simulink model "DiscreteSF_latest"  (R2019b)
settings: Solver=VariableStepAuto  StartTime=0.0  StopTime=1500  RelTol=1e-3
values from neighbouring files (symbols this model uses):
  A3 = [1 -49.59 4.877; 0 0.9835 0; 0 0 0.9512]    [DiscreteSystem.m]
  A3_c = [0 -th2 th4; 0 -1/th3 0; 0 0 -1/th5]    [DiscreteSystem.m]
  A5 = [1 -49.59 -0.4121 4.877 0.1209; 0 0.9835 0.01639 0 0; 0 0 0.9835 0 0 ... (first row only)    [DiscreteSystem.m]
  B3 = [0.85 -0.4144 0.1229; 0 0.01653 0; 0 0 0.04877]    [DiscreteSystem.m]
  B3_c = [th1 0 0; 0 1/th3 0; 0 0 1/th5]    [DiscreteSystem.m]
  B5 = [0.85 -0.002296 0.002032; 0 0.0001374 0; 0 0.01653 0; 0 0 0.001209 ... (first row only)    [DiscreteSystem.m]
  C3 = [1 0 0; 0 1 0; 0 0 1]    [DiscreteSystem.m]
  C3_c = [1 0 0; 0 1 0; 0 0 1]    [DiscreteSystem.m]
  C5 = [1 0 0 0 0; 0 1 0 0 0; 0 0 1 0 0; 0 0 0 1 0; 0 0 0 0 1]    [DiscreteSystem.m]
  D3 = [0 0 0; 0 0 0; 0 0 0]    [DiscreteSystem.m]
  D3_c = [0 0 0; 0 0 0; 0 0 0]    [DiscreteSystem.m]
  D5 = [0 0 0; 0 0 0; 0 0 0; 0 0 0; 0 0 0]    [DiscreteSystem.m]
  F3 = [k/th2 -k*th3 (k*th5*th4)/(th2)]    [DiscreteSystem.m]
  F5 = k*[1/th2 -th3 -th3 (th4*th5)/th2 (th4*th5)/th2]    [DiscreteSystem.m]
  L = [1.05; 0; 0; 0; 0]    [DiscreteSystem.m]
  th1 = 0.85    [DiscreteSystem.m]
  th2 = 50    [DiscreteSystem.m]
  th3 = 60    [DiscreteSystem.m]
undefined symbols (not defined in the file or in its folder): C
libraries: dspsrcs4 x3
settings Model: Creator=akshita_jain  LastModifiedBy=akshita_jain

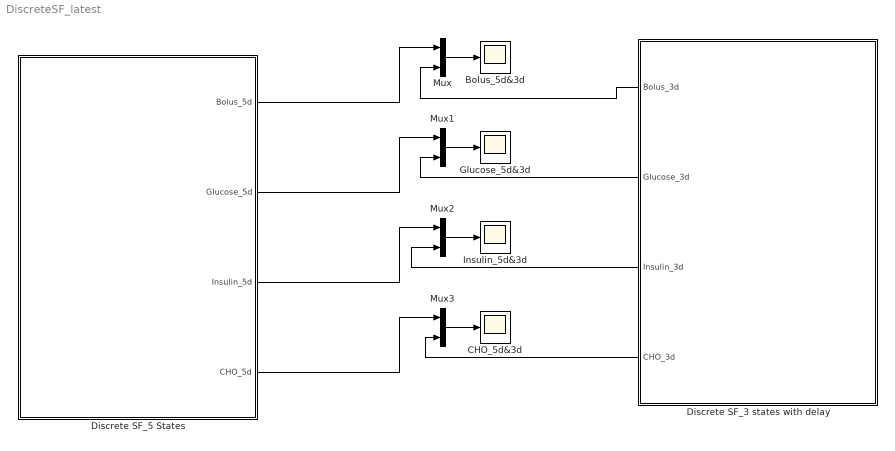
== system DiscreteSF_latest ==
  Bolus_5d&3d : Scope
  CHO_5d&3d : Scope
  Discrete SF_3 states with delay : Subsystem
  Discrete SF_5 States : Subsystem
  Glucose_5d&3d : Scope
  Insulin_5d&3d : Scope
  Mux{,1..3} (4 alike) : Mux  Inputs=2
  wires:
  Discrete SF_5 States/1(Bolus_5d) -> Mux/1
  Discrete SF_3 states with delay/1(Bolus_3d) -> Mux/2
  Mux/1 -> Bolus_5d&3d/1
  Mux1/1 -> Glucose_5d&3d/1
  Discrete SF_5 States/2(Glucose_5d) -> Mux1/1
  Discrete SF_3 states with delay/2(Glucose_3d) -> Mux1/2
  Mux2/1 -> Insulin_5d&3d/1
  Discrete SF_5 States/3(Insulin_5d) -> Mux2/1
  Discrete SF_3 states with delay/3(Insulin_3d) -> Mux2/2
  Discrete SF_5 States/4(CHO_5d) -> Mux3/1
  Mux3/1 -> CHO_5d&3d/1
  Discrete SF_3 states with delay/4(CHO_3d) -> Mux3/2

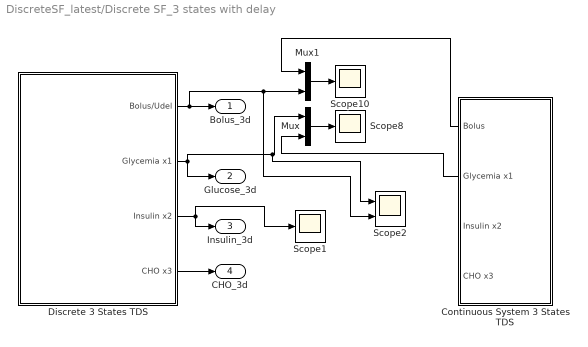
== system DiscreteSF_latest/Discrete SF_3 states with delay ==
  Continuous System 3 States TDS : Subsystem
  Discrete 3 States TDS : Subsystem
  Mux : Mux  Inputs=2
  Mux1 : Mux  Inputs=2
  Scope1 : Scope
  Scope10 : Scope
  Scope2 : Scope  NumInputPorts=2
  Scope8 : Scope
  Bolus_3d : Outport
  Glucose_3d : Outport  Port=2
  Insulin_3d : Outport  Port=3
  CHO_3d : Outport  Port=4
  wires:
  Discrete 3 States TDS/2(Glycemia x1) -> Glucose_3d/1, Scope2/1, Mux/1
  Discrete 3 States TDS/3(Insulin x2) -> Insulin_3d/1, Scope1/1
  Discrete 3 States TDS/4(CHO x3) -> CHO_3d/1
  Continuous System 3 States TDS/1(Bolus) -> Mux1/1
  Continuous System 3 States TDS/2(Glycemia x1) -> Mux/2
  Mux/1 -> Scope8/1
  Mux1/1 -> Scope10/1
  Discrete 3 States TDS/1(Bolus/Udel) -> Bolus_3d/1, Scope2/2, Mux1/2

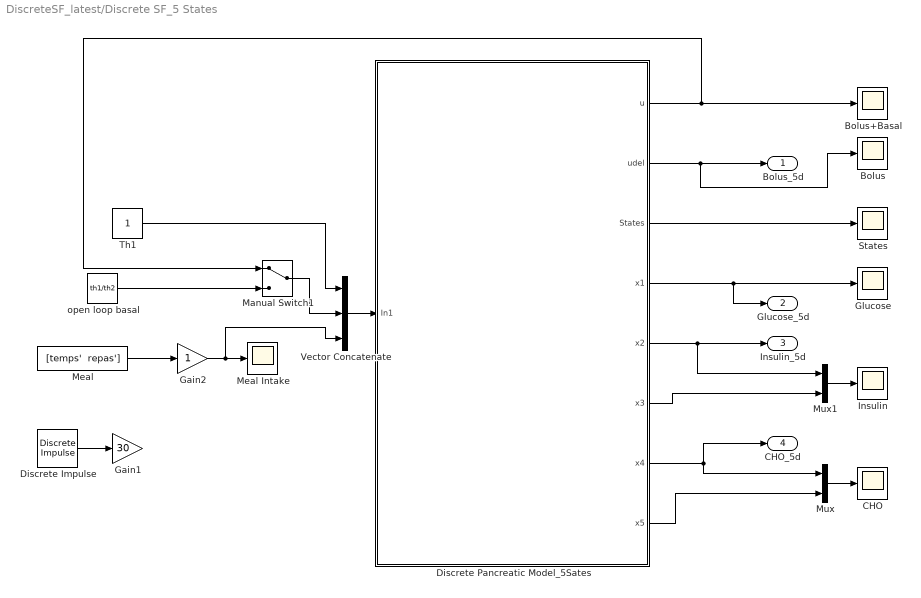
== system DiscreteSF_latest/Discrete SF_5 States ==
  Bolus : Scope
  Bolus+Basal : Scope
  CHO : Scope
  Discrete Impulse : dspsrcs4/Discrete  Impulse  Delay=110  SampleTime=1  FrameSample=1  OutputFrames=off  dataType=double  isSigned=on  wordLen=16  udDataType=sfix(16)  fracBitsMode=Best precision  numFracBits=15  OutDataTypeStr=double  LastOutDataTypeStr=double
  "Discrete Pancreatic Model_5Sates " : Subsystem
  Gain1 : Gain  Gain=30
  Gain2 : Gain
  Glucose : Scope
  Insulin : Scope
  Manual Switch1 : ManualSwitch
  Meal : FromWorkspace  VariableName="[temps'  repas']"  SampleTime=0
  Meal Intake : Scope
  Mux : Mux  Inputs=2
  Mux1 : Mux  Inputs=2
  States : Scope
  Th1 : Constant
  Vector Concatenate : Concatenate  NumInputs=3
  open loop basal : Constant  Value=th1/th2
  Bolus_5d : Outport
  Glucose_5d : Outport  Port=2
  Insulin_5d : Outport  Port=3
  CHO_5d : Outport  Port=4
  wires:
  "Discrete Pancreatic Model_5Sates "/2(udel) -> Bolus/1, Bolus_5d/1
  open loop basal/1 -> Manual Switch1/2
  Th1/1 -> Vector Concatenate/1
  Vector Concatenate/1 -> "Discrete Pancreatic Model_5Sates "/1(In1)
  "Discrete Pancreatic Model_5Sates "/3(States) -> States/1
  Discrete Impulse/1 -> Gain1/1
  "Discrete Pancreatic Model_5Sates "/7(x4) -> CHO_5d/1, Mux/1
  "Discrete Pancreatic Model_5Sates "/8(x5) -> Mux/2
  Mux/1 -> CHO/1
  "Discrete Pancreatic Model_5Sates "/6(x3) -> Mux1/2
  Mux1/1 -> Insulin/1
  "Discrete Pancreatic Model_5Sates "/4(x1) -> Glucose_5d/1, Glucose/1
  Gain2/1 -> Vector Concatenate/3, Meal Intake/1
  Meal/1 -> Gain2/1
  "Discrete Pancreatic Model_5Sates "/5(x2) -> Mux1/1, Insulin_5d/1
  "Discrete Pancreatic Model_5Sates "/1(u) -> Manual Switch1/1, Bolus+Basal/1
  Manual Switch1/1 -> Vector Concatenate/2

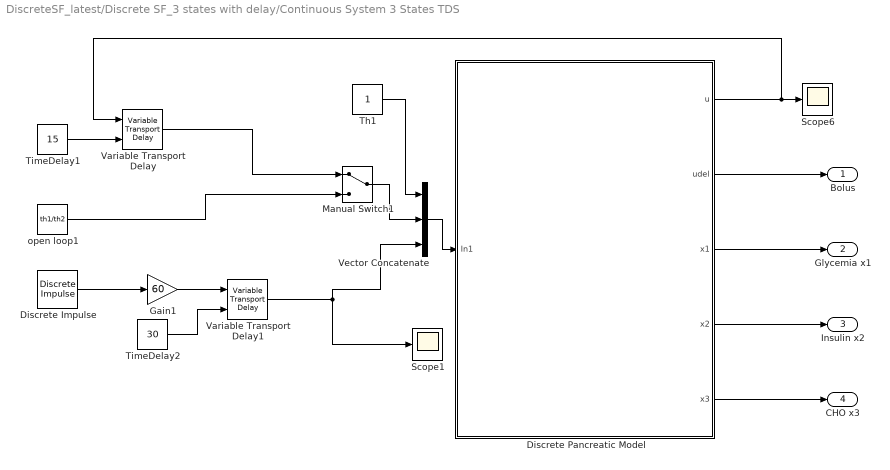
== system DiscreteSF_latest/Discrete SF_3 states with delay/Continuous System 3 States TDS ==
  Discrete Impulse : dspsrcs4/Discrete  Impulse  Delay=110  SampleTime=1  FrameSample=1  OutputFrames=off  dataType=double  isSigned=on  wordLen=16  udDataType=sfix(16)  fracBitsMode=Best precision  numFracBits=15  OutDataTypeStr=double  LastOutDataTypeStr=double
  Discrete Pancreatic Model : Subsystem
  Gain1 : Gain  Gain=60
  Manual Switch1 : ManualSwitch
  Scope1 : Scope
  Scope6 : Scope
  Th1 : Constant
  TimeDelay1 : Constant  Value=15
  TimeDelay2 : Constant  Value=30
  Variable Transport Delay : VariableTransportDelay  VariableDelayType=Variable transport delay  MaximumDelay=20  InitialOutput=th1/th2
  Variable Transport Delay1 : VariableTransportDelay  VariableDelayType=Variable transport delay  MaximumDelay=40
  Vector Concatenate : Concatenate  NumInputs=3
  open loop1 : Constant  Value=th1/th2
  Bolus : Outport
  Glycemia x1 : Outport  Port=2
  Insulin x2 : Outport  Port=3
  CHO x3 : Outport  Port=4
  wires:
  Discrete Pancreatic Model/3(x1) -> Glycemia x1/1
  Discrete Impulse/1 -> Gain1/1
  Vector Concatenate/1 -> Discrete Pancreatic Model/1(In1)
  Discrete Pancreatic Model/5(x3) -> CHO x3/1
  Discrete Pancreatic Model/4(x2) -> Insulin x2/1
  open loop1/1 -> Manual Switch1/2
  Variable Transport Delay/1 -> Manual Switch1/1
  Variable Transport Delay1/1 -> Vector Concatenate/3, Scope1/1
  Discrete Pancreatic Model/1(u) -> Variable Transport Delay/1, Scope6/1
  Gain1/1 -> Variable Transport Delay1/1
  Th1/1 -> Vector Concatenate/1
  Manual Switch1/1 -> Vector Concatenate/2
  Discrete Pancreatic Model/2(udel) -> Bolus/1
  TimeDelay1/1 -> Variable Transport Delay/2
  TimeDelay2/1 -> Variable Transport Delay1/2

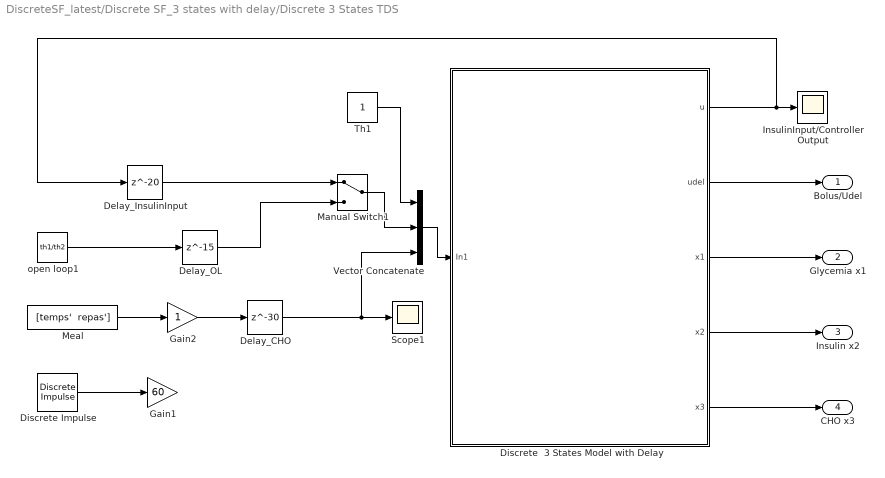
== system DiscreteSF_latest/Discrete SF_3 states with delay/Discrete 3 States TDS ==
  Delay_CHO : Delay  DelayLength=30  InitialCondition=0
  Delay_InsulinInput : Delay  DelayLength=20  InitialCondition=th1/th2
  Delay_OL : Delay  DelayLength=15  InitialCondition=th1/th2
  Discrete Impulse : dspsrcs4/Discrete  Impulse  Delay=110  SampleTime=1  FrameSample=1  OutputFrames=off  dataType=double  isSigned=on  wordLen=16  udDataType=sfix(16)  fracBitsMode=Best precision  numFracBits=15  OutDataTypeStr=double  LastOutDataTypeStr=double
  Discrete  3 States Model with Delay : Subsystem
  Gain1 : Gain  Gain=60
  Gain2 : Gain
  InsulinInput/ControllerOutput : Scope
  Manual Switch1 : ManualSwitch
  Meal : FromWorkspace  VariableName="[temps'  repas']"  SampleTime=0
  Scope1 : Scope
  Th1 : Constant
  Vector Concatenate : Concatenate  NumInputs=3
  open loop1 : Constant  Value=th1/th2
  Bolus/Udel : Outport
  Glycemia x1 : Outport  Port=2
  Insulin x2 : Outport  Port=3
  CHO x3 : Outport  Port=4
  wires:
  Discrete  3 States Model with Delay/3(x1) -> Glycemia x1/1
  Discrete Impulse/1 -> Gain1/1
  Vector Concatenate/1 -> Discrete  3 States Model with Delay/1(In1)
  Discrete  3 States Model with Delay/5(x3) -> CHO x3/1
  Discrete  3 States Model with Delay/4(x2) -> Insulin x2/1
  Delay_OL/1 -> Manual Switch1/2
  Delay_InsulinInput/1 -> Manual Switch1/1
  Delay_CHO/1 -> Vector Concatenate/3, Scope1/1
  Discrete  3 States Model with Delay/1(u) -> InsulinInput/ControllerOutput/1, Delay_InsulinInput/1
  Th1/1 -> Vector Concatenate/1
  Manual Switch1/1 -> Vector Concatenate/2
  Discrete  3 States Model with Delay/2(udel) -> Bolus/Udel/1
  open loop1/1 -> Delay_OL/1
  Meal/1 -> Gain2/1
  Gain2/1 -> Delay_CHO/1

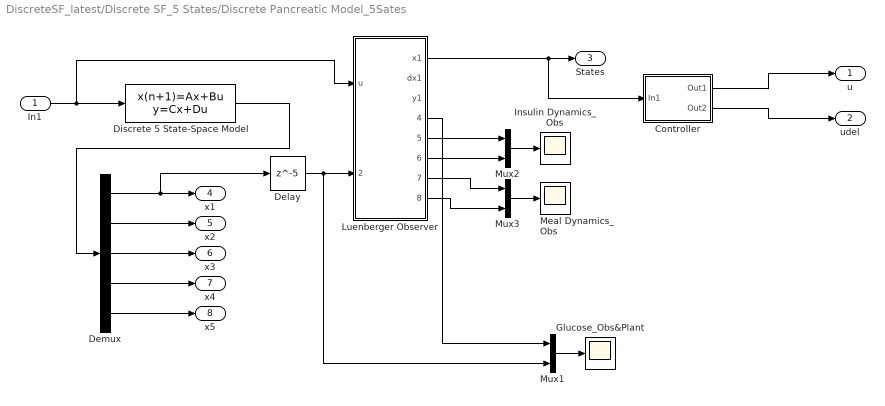
== system DiscreteSF_latest/Discrete SF_5 States/Discrete Pancreatic Model_5Sates  ==
  In1 : Inport
  Controller : Subsystem
  Delay : Delay  DelayLength=5  InitialCondition=110
  Demux : Demux  Outputs=5
  Discrete 5 State-Space Model : DiscreteStateSpace  A=A5  B=B5  C=C5  D=D5  InitialCondition=[110; th1/th2; th1/th2; 0; 0]  SampleTime=-1  StateName=Glycemia
  Glucose_Obs&Plant : Scope
  Insulin Dynamics_Obs : Scope
  Luenberger Observer : Subsystem
  Meal Dynamics_Obs : Scope
  Mux1 : Mux  Inputs=2
  Mux2 : Mux  Inputs=2
  Mux3 : Mux  Inputs=2
  u : Outport
  udel : Outport  Port=2
  States : Outport  Port=3
  x1 : Outport  Port=4
  x2 : Outport  Port=5
  x3 : Outport  Port=6
  x4 : Outport  Port=7
  x5 : Outport  Port=8
  wires:
  Discrete 5 State-Space Model/1 -> Demux/1
  In1/1 -> Luenberger Observer/1(u), Discrete 5 State-Space Model/1
  Demux/5 -> x5/1
  Demux/4 -> x4/1
  Demux/3 -> x3/1
  Demux/2 -> x2/1
  Luenberger Observer/1(x1) -> Controller/1(In1), States/1
  Mux1/1 -> Glucose_Obs&Plant/1
  Luenberger Observer/4(x1_obs) -> Mux1/1
  Mux2/1 -> Insulin Dynamics_Obs/1
  Luenberger Observer/5(x2_obs) -> Mux2/1
  Luenberger Observer/6(x3_obs) -> Mux2/2
  Luenberger Observer/8(x5_obs) -> Mux3/2
  Luenberger Observer/7(x4_obs) -> Mux3/1
  Mux3/1 -> Meal Dynamics_Obs/1
  Demux/1 -> Delay/1, x1/1
  Delay/1 -> Mux1/2, Luenberger Observer/2("y_plant ")
  Controller/1(Out1) -> u/1
  Controller/2(Out2) -> udel/1

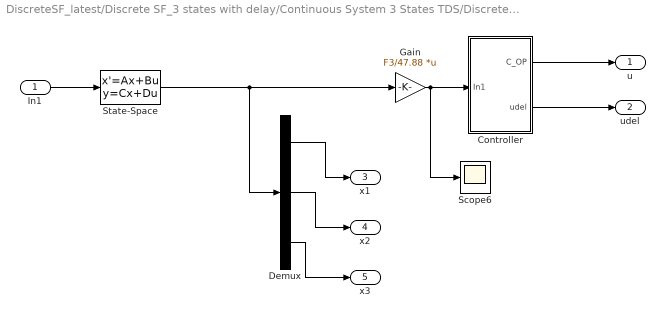
== system DiscreteSF_latest/Discrete SF_3 states with delay/Continuous System 3 States TDS/Discrete Pancreatic Model ==
  In1 : Inport
  "Controller " : Subsystem
  Demux : Demux  Outputs=3
  Gain : Gain  Gain=F3/47.88  Multiplication=Matrix(K*u)
  Scope6 : Scope
  State-Space : StateSpace  A=A3_c  B=B3_c  C=C3_c  D=D3_c  InitialCondition=[110; th1/th2; 0]
  u : Outport
  udel : Outport  Port=2
  x1 : Outport  Port=3
  x2 : Outport  Port=4
  x3 : Outport  Port=5
  wires:
  "Controller "/1(C_OP) -> u/1
  "Controller "/2(udel) -> udel/1
  State-Space/1 -> Demux/1, Gain/1
  Gain/1 -> Scope6/1, "Controller "/1(In1)
  In1/1 -> State-Space/1
  Demux/1 -> x1/1
  Demux/3 -> x3/1
  Demux/2 -> x2/1

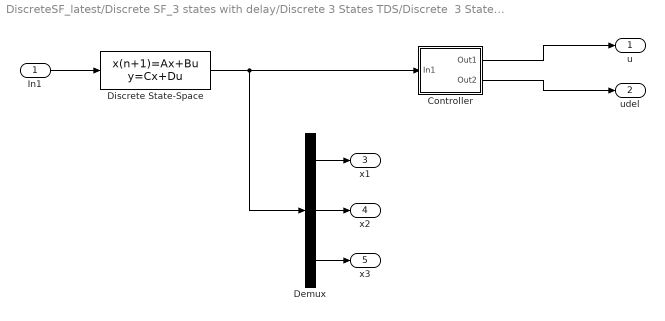
== system DiscreteSF_latest/Discrete SF_3 states with delay/Discrete 3 States TDS/Discrete  3 States Model with Delay ==
  In1 : Inport
  Controller : Subsystem
  Demux : Demux  Outputs=3
  Discrete State-Space : DiscreteStateSpace  A=A3  B=B3  C=C3  D=D3  InitialCondition=[110; th1/th2; 0]  SampleTime=-1  StateName=Glycemia
  u : Outport
  udel : Outport  Port=2
  x1 : Outport  Port=3
  x2 : Outport  Port=4
  x3 : Outport  Port=5
  wires:
  Discrete State-Space/1 -> Controller/1(In1), Demux/1
  In1/1 -> Discrete State-Space/1
  Demux/1 -> x1/1
  Demux/3 -> x3/1
  Demux/2 -> x2/1
  Controller/1(Out1) -> u/1
  Controller/2(Out2) -> udel/1

== system DiscreteSF_latest/Discrete SF_5 States/Discrete Pancreatic Model_5Sates /Controller ==
  In1 : Inport
  C1 : Subsystem
  Gain : Gain  Gain=F5*0.02  Multiplication=Matrix(K*u)
  Out1 : Outport
  Out2 : Outport  Port=2
  wires:
  C1/2(udel) -> Out2/1
  C1/1(C_OP) -> Out1/1
  In1/1 -> Gain/1
  Gain/1 -> C1/1(In1)

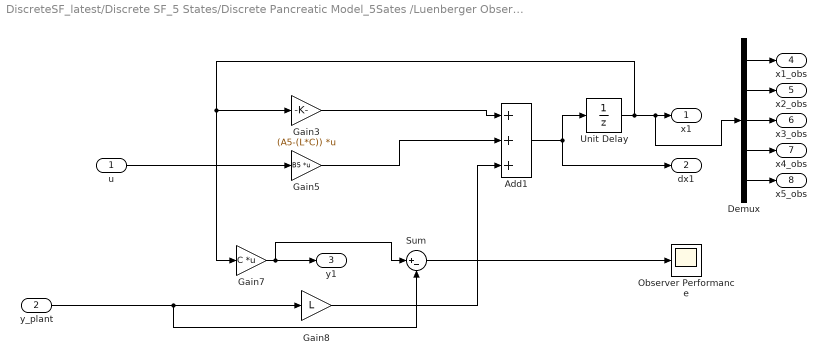
== system DiscreteSF_latest/Discrete SF_5 States/Discrete Pancreatic Model_5Sates /Luenberger Observer ==
  u : Inport
  "y_plant " : Inport  Port=2
  Add1 : Sum  Inputs=3
  Demux : Demux  Outputs=5
  Gain3 : Gain  Gain=(A5-(L*C))  Multiplication=Matrix(K*u)
  Gain5 : Gain  Gain=B5  Multiplication=Matrix(K*u)
  Gain7 : Gain  Gain=C  Multiplication=Matrix(K*u)
  Gain8 : Gain  Gain=L
  Observer Performance : Scope
  Sum : Sum  Inputs=|+-
  Unit Delay : UnitDelay  InitialCondition=[115; th1/th2; th1/th2; 0; 0]  SampleTime=-1  HasFrameUpgradeWarning=on
  x1 : Outport
  dx1 : Outport  Port=2
  y1 : Outport  Port=3
  x1_obs : Outport  Port=4
  x2_obs : Outport  Port=5
  x3_obs : Outport  Port=6
  x4_obs : Outport  Port=7
  x5_obs : Outport  Port=8
  wires:
  u/1 -> Gain5/1
  Sum/1 -> Observer Performance/1
  Add1/1 -> Unit Delay/1, dx1/1
  Unit Delay/1 -> Demux/1, x1/1, Gain3/1, Gain7/1
  Gain3/1 -> Add1/1
  Gain8/1 -> Add1/3
  Gain7/1 -> y1/1, Sum/1
  Demux/4 -> x4_obs/1
  Demux/2 -> x2_obs/1
  Demux/3 -> x3_obs/1
  Demux/5 -> x5_obs/1
  Demux/1 -> x1_obs/1
  "y_plant "/1 -> Sum/2, Gain8/1
  Gain5/1 -> Add1/2

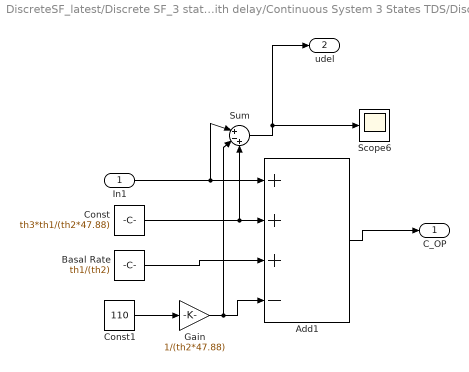
== system DiscreteSF_latest/Discrete SF_3 states with delay/Continuous System 3 States TDS/Discrete Pancreatic Model/Controller  ==
  In1 : Inport
  Add1 : Sum  Inputs=+++-
  Basal Rate : Constant  Value=th1/(th2)  VectorParams1D=off
  Const : Constant  Value=th3*th1/(th2*47.88)  VectorParams1D=off
  Const1 : Constant  Value=110  VectorParams1D=off
  Gain : Gain  Gain=1/(th2*47.88)
  Scope6 : Scope
  Sum : Sum  Inputs=|+-+
  C_OP : Outport
  udel : Outport  Port=2
  wires:
  Const/1 -> Sum/3, Add1/2
  Basal Rate/1 -> Add1/3
  Add1/1 -> C_OP/1
  Sum/1 -> Scope6/1, udel/1
  In1/1 -> Sum/1, Add1/1
  Const1/1 -> Gain/1
  Gain/1 -> Sum/2, Add1/4

== system DiscreteSF_latest/Discrete SF_3 states with delay/Discrete 3 States TDS/Discrete  3 States Model with Delay/Controller ==
  In1 : Inport
  "C1 " : Subsystem
  Gain : Gain  Gain=F3*0.022  Multiplication=Matrix(K*u)
  Out1 : Outport
  Out2 : Outport  Port=2
  wires:
  In1/1 -> Gain/1
  "C1 "/1(C_OP) -> Out1/1
  "C1 "/2(udel) -> Out2/1
  Gain/1 -> "C1 "/1(In1)

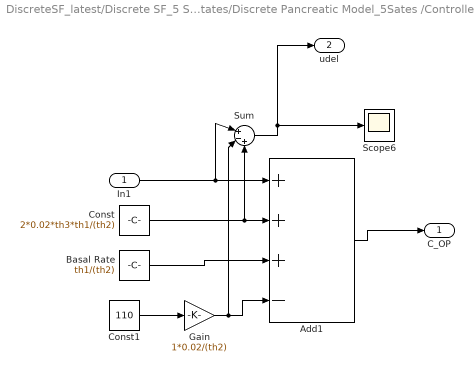
== system DiscreteSF_latest/Discrete SF_5 States/Discrete Pancreatic Model_5Sates /Controller/C1 ==
  In1 : Inport
  Add1 : Sum  Inputs=+++-
  Basal Rate : Constant  Value=th1/(th2)  VectorParams1D=off
  Const : Constant  Value=2*0.02*th3*th1/(th2)  VectorParams1D=off
  Const1 : Constant  Value=110  VectorParams1D=off
  Gain : Gain  Gain=1*0.02/(th2)
  Scope6 : Scope
  Sum : Sum  Inputs=|+-+
  C_OP : Outport
  udel : Outport  Port=2
  wires:
  Const/1 -> Sum/3, Add1/2
  Basal Rate/1 -> Add1/3
  Add1/1 -> C_OP/1
  Sum/1 -> Scope6/1, udel/1
  In1/1 -> Sum/1, Add1/1
  Const1/1 -> Gain/1
  Gain/1 -> Sum/2, Add1/4

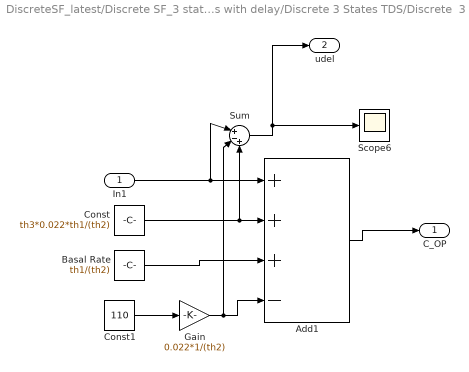
== system DiscreteSF_latest/Discrete SF_3 states with delay/Discrete 3 States TDS/Discrete  3 States Model with Delay/Controller/C1  ==
  In1 : Inport
  Add1 : Sum  Inputs=+++-
  Basal Rate : Constant  Value=th1/(th2)  VectorParams1D=off
  Const : Constant  Value=th3*0.022*th1/(th2)  VectorParams1D=off
  Const1 : Constant  Value=110  VectorParams1D=off
  Gain : Gain  Gain=0.022*1/(th2)
  Scope6 : Scope
  Sum : Sum  Inputs=|+-+
  C_OP : Outport
  udel : Outport  Port=2
  wires:
  Const/1 -> Sum/3, Add1/2
  Basal Rate/1 -> Add1/3
  Add1/1 -> C_OP/1
  Sum/1 -> Scope6/1, udel/1
  In1/1 -> Sum/1, Add1/1
  Const1/1 -> Gain/1
  Gain/1 -> Sum/2, Add1/4
